simulink model "Hydraulic787"  (R2013a)
settings: Solver=ode23tb  StartTime=0.0  StopTime=1000  RelTol=1e-3
InitFcn:
  | load('SampleOutput.mat')
  | 
  | load('SampleFuelBurn.mat')
undefined symbols (not defined in the file): ailerons, AirProp, B_737, elevator, HydProp, landing_gear, rudder, thrust_rev
libraries: PowerFlowLib x43, simulink x4
(part 2 of 2)

== system Hydraulic787/Center Hydraulic System/DC Speed Servo1 ==
  T_load (Nm) : Inport
  Speed_ref (RPM) : Inport  Port=2
  Voltage : Inport  Port=3
  DC Machine : Subsystem
  Fcn : Fcn  Expr=u(1)/(u(2)+0.1)
  Gain2 : Gain  Gain=60/(2*pi)
  Mux : Mux  Inputs=2
  PID Controller : simulink/Continuous/PID Controller  Controller=PID  TimeDomain=Continuous-time  SampleTime=1  IntegratorMethod=Forward Euler  FilterMethod=Forward Euler  Form=Parallel  P=1  I=0.1  D=0  N=100  InitialConditionSource=internal  InitialConditionForIntegrator=0  InitialConditionForFilter=0  ExternalReset=none  LimitOutput=off  UpperSaturationLimit=inf  LowerSaturationLimit=-inf  LinearizeAsGain=on  AntiWindupMode=none  Kb=1  TrackingMode=off  Kt=1  PParamMin=[]  PParamMax=[]  IParamMin=[]  IParamMax=[]  DParamMin=[]  DParamMax=[]  NParamMin=[]  NParamMax=[]  KbParamMin=[]  KbParamMax=[]  KtParamMin=[]  KtParamMax=[]  POutMin=[]  POutMax=[]  IOutMin=[]  IOutMax=[]  DOutMin=[]  DOutMax=[]  NOutMin=[]  NOutMax=[]  KbOutMin=[]  KbOutMax=[]  KtOutMin=[]  KtOutMax=[]  IntegratorOutMin=[]  IntegratorOutMax=[]  FilterOutMin=[]  FilterOutMax=[]  SumOutMin=[]  SumOutMax=[]  SumI1OutMin=[]  SumI1OutMax=[]  SumI2OutMin=[]  SumI2OutMax=[]  SumI3OutMin=[]  SumI3OutMax=[]  SumDOutMin=[]  SumDOutMax=[]  SaturationOutMin=[]  SaturationOutMax=[]  IntegratorContinuousStateAttributes=''  IntegratorStateMustResolveToSignalObject=off  IntegratorRTWStateStorageClass=Auto  FilterContinuousStateAttributes=''  FilterStateMustResolveToSignalObject=off  FilterRTWStateStorageClass=Auto
  Sum : Sum  Inputs=-+|
  Terminator{,1..3} (4 alike) : Terminator
  w_m : Outport
  i_load : Outport  Port=2
  T_em : Outport  Port=3
  Ploss : Outport  Port=4
  wires:
  DC Machine/5(Plosses) -> Ploss/1
  Sum/1 -> PID Controller/1
  Gain2/1 -> Sum/1, w_m/1
  Speed_ref (RPM)/1 -> Sum/2
  T_load (Nm)/1 -> DC Machine/3(Tload)
  DC Machine/6(Te) -> T_em/1
  Mux/1 -> Fcn/1
  DC Machine/3(Pe) -> Mux/1
  Fcn/1 -> i_load/1
  DC Machine/7(Speed) -> Gain2/1
  Voltage/1 -> DC Machine/1(Vf), Mux/2
  PID Controller/1 -> DC Machine/2(Va)
  DC Machine/1(If) -> Terminator3/1
  DC Machine/2(Ia) -> Terminator2/1
  DC Machine/4(Pm) -> Terminator1/1
  DC Machine/8(theta) -> Terminator/1

== system Hydraulic787/Center Hydraulic System/Sinks ==
  "Motor PLoss 1 " : Inport
  Motor PLoss 2 : Inport  Port=2
  Motor Current Load 1 : Inport  Port=3
  Motor Current Load 2 : Inport  Port=4
  Out1 : Outport
  wires:
  "Motor PLoss 1 "/1 -> Out1/1

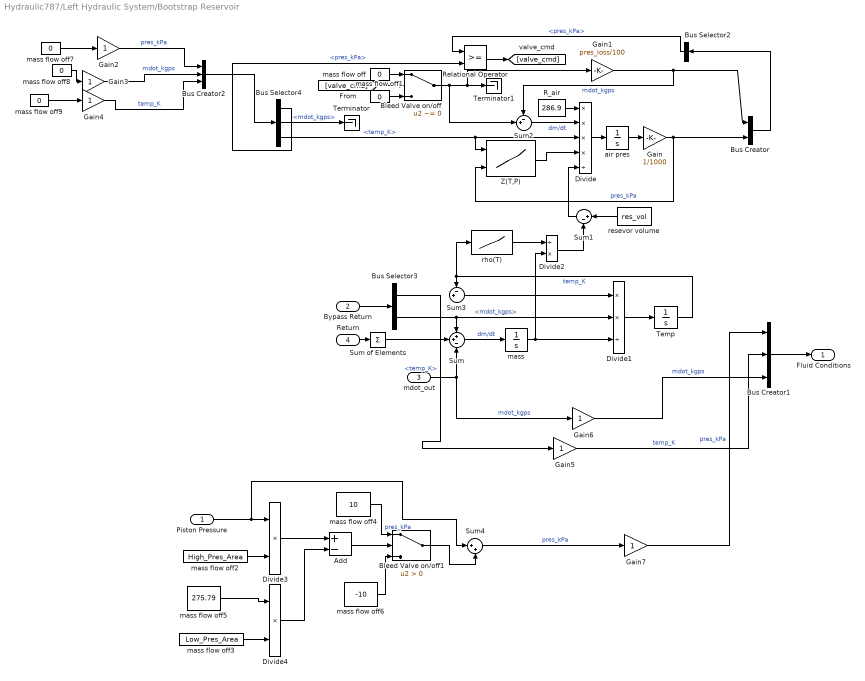
== system Hydraulic787/Left Hydraulic System/Bootstrap Reservoir ==
  Piston Pressure : Inport
  Bypass Return : Inport  Port=2
  mdot_out : Inport  Port=3
  Return : Inport  Port=4
  Add : Sum  Inputs=+-
  Bleed Valve on/off : Switch  Criteria=u2 ~= 0  ZeroCross=off
  Bleed Valve on/off1 : Switch  Criteria=u2 > Threshold  ZeroCross=off
  Bus Creator : BusCreator  Inputs=2
  Bus Creator1 : BusCreator  Inputs=3
  Bus Creator2 : BusCreator  Inputs=3
  Bus Selector2 : BusSelector  OutputSignals=pres_kPa
  Bus Selector3 : BusSelector  OutputSignals=temp_K,mdot_kgps
  Bus Selector4 : BusSelector  OutputSignals=pres_kPa,mdot_kgps,temp_K
  Divide : Product  Inputs=****/
  Divide1 : Product  Inputs=**/
  Divide2 : Product  Inputs=/*
  Divide3 : Product  Inputs=**
  Divide4 : Product  Inputs=**
  Gain : Gain  Gain=1/1000
  Gain1 : Gain  Gain=pres_loss/100
  Gain{2..7} (6 alike) : Gain
  R_air : Constant  Value=286.9
  Relational Operator : RelationalOperator  OutDataTypeStr=boolean
  Sum : Sum  Inputs=++-
  Sum of Elements : Sum  Inputs=+
  Sum1 : Sum  Inputs=|+-
  Sum2 : Sum  Inputs=-+|
  Sum3 : Sum  Inputs=-+|
  Sum4 : Sum  Inputs=|++
  Temp : Integrator  InitialCondition=T_init  LimitOutput=on  LowerSaturationLimit=eps
  Terminator : Terminator
  Terminator1 : Terminator
  Z(T,P) : Lookup_n-D  BreakpointsForDimension1=AirProp.T2  BreakpointsForDimension2=AirProp.P2  Table=AirProp.Z  RndMeth=Simplest  InputSameDT=on
  air pres : Integrator  InitialCondition=P_init*1000
  mass : Integrator  InitialCondition=mass_init  LimitOutput=on  LowerSaturationLimit=eps
  mass flow off{,1,7..9} (5 alike) : Constant  Value=0
  mass flow off2 : Constant  Value=High_Pres_Area
  mass flow off3 : Constant  Value=Low_Pres_Area
  mass flow off4 : Constant  Value=10
  mass flow off5 : Constant  Value=275.79
  mass flow off6 : Constant  Value=-10
  resevor volume : Constant  Value=res_vol
  rho(T) : Lookup_n-D  NumberOfTableDimensions=1  BreakpointsForDimension1=HydProp.T  Table=HydProp.rho_T  RndMeth=Simplest  InputSameDT=on
  Fluid Conditions : Outport
  wires:
  Piston Pressure/1 -> Sum4/1, Divide3/1
  mass flow off1/1 -> Bleed Valve on/off/3
  Divide2/1 -> Sum1/2
  rho(T)/1 -> Divide2/1
  Sum of Elements/1 -> Sum/2
  Return/1 -> Sum of Elements/1
  Bus Selector3/1 -> Gain5/1  "<temp_K>"
  Temp/1 -> rho(T)/1, Sum3/1  "temp_K"
  Sum3/1 -> Divide1/1
  Divide1/1 -> Temp/1
  mass/1 -> Divide1/3, Divide2/2
  Bus Creator1/1 -> Fluid Conditions/1
  [valve_cmd] -> Bleed Valve on/off/2
  Relational Operator/1 -> [valve_cmd]
  mass flow off/1 -> Bleed Valve on/off/1
  Bus Selector2/1 -> Relational Operator/1  "<pres_kPa>"
  Bus Selector4/1 -> Relational Operator/2  "<pres_kPa>"
  Bleed Valve on/off/1 -> Terminator1/1, Gain1/1, Sum2/2
  Bus Selector4/2 -> Terminator/1  "<mdot_kgps>"
  Sum2/1 -> Divide/2  "dm/dt"
  Bus Creator/1 -> Bus Selector2/1
  Gain1/1 -> Sum2/1, Bus Creator/1  "mdot_kgps"
  Gain/1 -> Bus Creator/2, Z(T,P)/2  "pres_kPa"
  Sum1/1 -> Divide/5
  resevor volume/1 -> Sum1/1
  air pres/1 -> Gain/1
  Divide/1 -> air pres/1
  Z(T,P)/1 -> Divide/4
  R_air/1 -> Divide/1
  Bus Selector4/3 -> Divide/3, Z(T,P)/1  "<temp_K>"
  Sum/1 -> mass/1  "dm/dt"
  mdot_out/1 -> Gain6/1, Sum/3  "mdot_kgps"
  Bus Selector3/2 -> Sum/1, Divide1/2  "<mdot_kgps>"
  Bypass Return/1 -> Bus Selector3/1
  mass flow off2/1 -> Divide3/2
  mass flow off3/1 -> Divide4/2
  mass flow off5/1 -> Divide4/1
  Divide4/1 -> Add/2
  Divide3/1 -> Add/1
  Add/1 -> Bleed Valve on/off1/2
  mass flow off6/1 -> Bleed Valve on/off1/3
  Bleed Valve on/off1/1 -> Sum4/2
  mass flow off4/1 -> Bleed Valve on/off1/1  "pres_kPa"
  Bus Creator2/1 -> Bus Selector4/1
  mass flow off9/1 -> Gain4/1
  mass flow off8/1 -> Gain3/1
  mass flow off7/1 -> Gain2/1
  Gain2/1 -> Bus Creator2/1  "pres_kPa"
  Gain4/1 -> Bus Creator2/3  "temp_K"
  Gain3/1 -> Bus Creator2/2  "mdot_kgps"
  Gain7/1 -> Bus Creator1/1  "pres_kPa"
  Gain6/1 -> Bus Creator1/3  "mdot_kgps"
  Gain5/1 -> Bus Creator1/2  "temp_K"
  Sum4/1 -> Gain7/1  "pres_kPa"

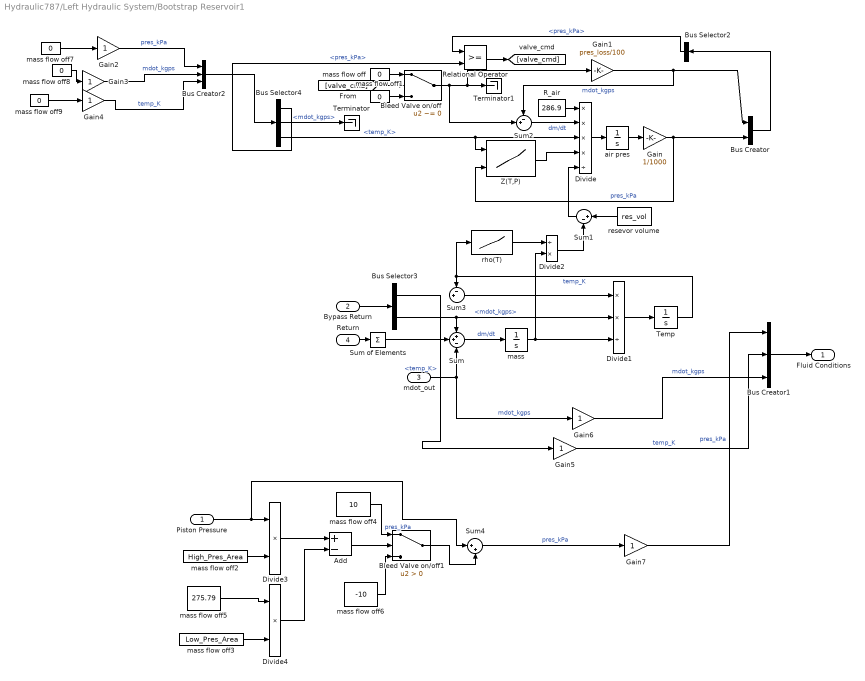
== system Hydraulic787/Left Hydraulic System/Bootstrap Reservoir1 ==
  Piston Pressure : Inport
  Bypass Return : Inport  Port=2
  mdot_out : Inport  Port=3
  Return : Inport  Port=4
  Add : Sum  Inputs=+-
  Bleed Valve on/off : Switch  Criteria=u2 ~= 0  ZeroCross=off
  Bleed Valve on/off1 : Switch  Criteria=u2 > Threshold  ZeroCross=off
  Bus Creator : BusCreator  Inputs=2
  Bus Creator1 : BusCreator  Inputs=3
  Bus Creator2 : BusCreator  Inputs=3
  Bus Selector2 : BusSelector  OutputSignals=pres_kPa
  Bus Selector3 : BusSelector  OutputSignals=temp_K,mdot_kgps
  Bus Selector4 : BusSelector  OutputSignals=pres_kPa,mdot_kgps,temp_K
  Divide : Product  Inputs=****/
  Divide1 : Product  Inputs=**/
  Divide2 : Product  Inputs=/*
  Divide3 : Product  Inputs=**
  Divide4 : Product  Inputs=**
  Gain : Gain  Gain=1/1000
  Gain1 : Gain  Gain=pres_loss/100
  Gain{2..7} (6 alike) : Gain
  R_air : Constant  Value=286.9
  Relational Operator : RelationalOperator  OutDataTypeStr=boolean
  Sum : Sum  Inputs=++-
  Sum of Elements : Sum  Inputs=+
  Sum1 : Sum  Inputs=|+-
  Sum2 : Sum  Inputs=-+|
  Sum3 : Sum  Inputs=-+|
  Sum4 : Sum  Inputs=|++
  Temp : Integrator  InitialCondition=T_init  LimitOutput=on  LowerSaturationLimit=eps
  Terminator : Terminator
  Terminator1 : Terminator
  Z(T,P) : Lookup_n-D  BreakpointsForDimension1=AirProp.T2  BreakpointsForDimension2=AirProp.P2  Table=AirProp.Z  RndMeth=Simplest  InputSameDT=on
  air pres : Integrator  InitialCondition=P_init*1000
  mass : Integrator  InitialCondition=mass_init  LimitOutput=on  LowerSaturationLimit=eps
  mass flow off{,1,7..9} (5 alike) : Constant  Value=0
  mass flow off2 : Constant  Value=High_Pres_Area
  mass flow off3 : Constant  Value=Low_Pres_Area
  mass flow off4 : Constant  Value=10
  mass flow off5 : Constant  Value=275.79
  mass flow off6 : Constant  Value=-10
  resevor volume : Constant  Value=res_vol
  rho(T) : Lookup_n-D  NumberOfTableDimensions=1  BreakpointsForDimension1=HydProp.T  Table=HydProp.rho_T  RndMeth=Simplest  InputSameDT=on
  Fluid Conditions : Outport
  wires:
  Piston Pressure/1 -> Sum4/1, Divide3/1
  mass flow off1/1 -> Bleed Valve on/off/3
  Divide2/1 -> Sum1/2
  rho(T)/1 -> Divide2/1
  Sum of Elements/1 -> Sum/2
  Return/1 -> Sum of Elements/1
  Bus Selector3/1 -> Gain5/1  "<temp_K>"
  Temp/1 -> rho(T)/1, Sum3/1  "temp_K"
  Sum3/1 -> Divide1/1
  Divide1/1 -> Temp/1
  mass/1 -> Divide1/3, Divide2/2
  Bus Creator1/1 -> Fluid Conditions/1
  [valve_cmd] -> Bleed Valve on/off/2
  Relational Operator/1 -> [valve_cmd]
  mass flow off/1 -> Bleed Valve on/off/1
  Bus Selector2/1 -> Relational Operator/1  "<pres_kPa>"
  Bus Selector4/1 -> Relational Operator/2  "<pres_kPa>"
  Bleed Valve on/off/1 -> Terminator1/1, Gain1/1, Sum2/2
  Bus Selector4/2 -> Terminator/1  "<mdot_kgps>"
  Sum2/1 -> Divide/2  "dm/dt"
  Bus Creator/1 -> Bus Selector2/1
  Gain1/1 -> Sum2/1, Bus Creator/1  "mdot_kgps"
  Gain/1 -> Bus Creator/2, Z(T,P)/2  "pres_kPa"
  Sum1/1 -> Divide/5
  resevor volume/1 -> Sum1/1
  air pres/1 -> Gain/1
  Divide/1 -> air pres/1
  Z(T,P)/1 -> Divide/4
  R_air/1 -> Divide/1
  Bus Selector4/3 -> Divide/3, Z(T,P)/1  "<temp_K>"
  Sum/1 -> mass/1  "dm/dt"
  mdot_out/1 -> Gain6/1, Sum/3  "mdot_kgps"
  Bus Selector3/2 -> Sum/1, Divide1/2  "<mdot_kgps>"
  Bypass Return/1 -> Bus Selector3/1
  mass flow off2/1 -> Divide3/2
  mass flow off3/1 -> Divide4/2
  mass flow off5/1 -> Divide4/1
  Divide4/1 -> Add/2
  Divide3/1 -> Add/1
  Add/1 -> Bleed Valve on/off1/2
  mass flow off6/1 -> Bleed Valve on/off1/3
  Bleed Valve on/off1/1 -> Sum4/2
  mass flow off4/1 -> Bleed Valve on/off1/1  "pres_kPa"
  Bus Creator2/1 -> Bus Selector4/1
  mass flow off9/1 -> Gain4/1
  mass flow off8/1 -> Gain3/1
  mass flow off7/1 -> Gain2/1
  Gain2/1 -> Bus Creator2/1  "pres_kPa"
  Gain4/1 -> Bus Creator2/3  "temp_K"
  Gain3/1 -> Bus Creator2/2  "mdot_kgps"
  Gain7/1 -> Bus Creator1/1  "pres_kPa"
  Gain6/1 -> Bus Creator1/3  "mdot_kgps"
  Gain5/1 -> Bus Creator1/2  "temp_K"
  Sum4/1 -> Gain7/1  "pres_kPa"

== system Hydraulic787/Left Hydraulic System/DC Speed Servo ==
  T_load (Nm) : Inport
  Speed_ref (RPM) : Inport  Port=2
  Voltage : Inport  Port=3
  DC Machine : Subsystem
  Fcn : Fcn  Expr=u(1)/(u(2)+0.1)
  Gain2 : Gain  Gain=60/(2*pi)
  Mux : Mux  Inputs=2
  PID Controller : simulink/Continuous/PID Controller  Controller=PID  TimeDomain=Continuous-time  SampleTime=1  IntegratorMethod=Forward Euler  FilterMethod=Forward Euler  Form=Parallel  P=1  I=0.1  D=0  N=100  InitialConditionSource=internal  InitialConditionForIntegrator=0  InitialConditionForFilter=0  ExternalReset=none  LimitOutput=off  UpperSaturationLimit=inf  LowerSaturationLimit=-inf  LinearizeAsGain=on  AntiWindupMode=none  Kb=1  TrackingMode=off  Kt=1  PParamMin=[]  PParamMax=[]  IParamMin=[]  IParamMax=[]  DParamMin=[]  DParamMax=[]  NParamMin=[]  NParamMax=[]  KbParamMin=[]  KbParamMax=[]  KtParamMin=[]  KtParamMax=[]  POutMin=[]  POutMax=[]  IOutMin=[]  IOutMax=[]  DOutMin=[]  DOutMax=[]  NOutMin=[]  NOutMax=[]  KbOutMin=[]  KbOutMax=[]  KtOutMin=[]  KtOutMax=[]  IntegratorOutMin=[]  IntegratorOutMax=[]  FilterOutMin=[]  FilterOutMax=[]  SumOutMin=[]  SumOutMax=[]  SumI1OutMin=[]  SumI1OutMax=[]  SumI2OutMin=[]  SumI2OutMax=[]  SumI3OutMin=[]  SumI3OutMax=[]  SumDOutMin=[]  SumDOutMax=[]  SaturationOutMin=[]  SaturationOutMax=[]  IntegratorContinuousStateAttributes=''  IntegratorStateMustResolveToSignalObject=off  IntegratorRTWStateStorageClass=Auto  FilterContinuousStateAttributes=''  FilterStateMustResolveToSignalObject=off  FilterRTWStateStorageClass=Auto
  Sum : Sum  Inputs=-+|
  Terminator{,1..3} (4 alike) : Terminator
  w_m : Outport
  i_load : Outport  Port=2
  T_em : Outport  Port=3
  Ploss : Outport  Port=4
  wires:
  DC Machine/5(Plosses) -> Ploss/1
  Sum/1 -> PID Controller/1
  Gain2/1 -> Sum/1, w_m/1
  Speed_ref (RPM)/1 -> Sum/2
  T_load (Nm)/1 -> DC Machine/3(Tload)
  DC Machine/6(Te) -> T_em/1
  Mux/1 -> Fcn/1
  DC Machine/3(Pe) -> Mux/1
  Fcn/1 -> i_load/1
  DC Machine/7(Speed) -> Gain2/1
  Voltage/1 -> DC Machine/1(Vf), Mux/2
  PID Controller/1 -> DC Machine/2(Va)
  DC Machine/1(If) -> Terminator/1
  DC Machine/2(Ia) -> Terminator1/1
  DC Machine/4(Pm) -> Terminator2/1
  DC Machine/8(theta) -> Terminator3/1

== system Hydraulic787/Left Hydraulic System/Sinks ==
  "Motor PLoss " : Inport
  Motor Current Load : Inport  Port=2
  Out1 : Outport
  wires:
  "Motor PLoss "/1 -> Out1/1

== system Hydraulic787/Right Hydraulic System/Bootstrap Reservoir ==
  Piston Pressure : Inport
  Bypass Return : Inport  Port=2
  mdot_out : Inport  Port=3
  Return : Inport  Port=4
  Add : Sum  Inputs=+-
  Bleed Valve on/off : Switch  Criteria=u2 ~= 0  ZeroCross=off
  Bleed Valve on/off1 : Switch  Criteria=u2 > Threshold  ZeroCross=off
  Bus Creator : BusCreator  Inputs=2
  Bus Creator1 : BusCreator  Inputs=3
  Bus Creator2 : BusCreator  Inputs=3
  Bus Selector2 : BusSelector  OutputSignals=pres_kPa
  Bus Selector3 : BusSelector  OutputSignals=temp_K,mdot_kgps
  Bus Selector4 : BusSelector  OutputSignals=pres_kPa,mdot_kgps,temp_K
  Divide : Product  Inputs=****/
  Divide1 : Product  Inputs=**/
  Divide2 : Product  Inputs=/*
  Divide3 : Product  Inputs=**
  Divide4 : Product  Inputs=**
  Gain : Gain  Gain=1/1000
  Gain1 : Gain  Gain=pres_loss/100
  Gain{2..7} (6 alike) : Gain
  R_air : Constant  Value=286.9
  Relational Operator : RelationalOperator  OutDataTypeStr=boolean
  Sum : Sum  Inputs=++-
  Sum of Elements : Sum  Inputs=+
  Sum1 : Sum  Inputs=|+-
  Sum2 : Sum  Inputs=-+|
  Sum3 : Sum  Inputs=-+|
  Sum4 : Sum  Inputs=|++
  Temp : Integrator  InitialCondition=T_init  LimitOutput=on  LowerSaturationLimit=eps
  Terminator : Terminator
  Terminator1 : Terminator
  Z(T,P) : Lookup_n-D  BreakpointsForDimension1=AirProp.T2  BreakpointsForDimension2=AirProp.P2  Table=AirProp.Z  RndMeth=Simplest  InputSameDT=on
  air pres : Integrator  InitialCondition=P_init*1000
  mass : Integrator  InitialCondition=mass_init  LimitOutput=on  LowerSaturationLimit=eps
  mass flow off{,1,7..9} (5 alike) : Constant  Value=0
  mass flow off2 : Constant  Value=High_Pres_Area
  mass flow off3 : Constant  Value=Low_Pres_Area
  mass flow off4 : Constant  Value=10
  mass flow off5 : Constant  Value=275.79
  mass flow off6 : Constant  Value=-10
  resevor volume : Constant  Value=res_vol
  rho(T) : Lookup_n-D  NumberOfTableDimensions=1  BreakpointsForDimension1=HydProp.T  Table=HydProp.rho_T  RndMeth=Simplest  InputSameDT=on
  Fluid Conditions : Outport
  wires:
  Piston Pressure/1 -> Sum4/1, Divide3/1
  mass flow off1/1 -> Bleed Valve on/off/3
  Divide2/1 -> Sum1/2
  rho(T)/1 -> Divide2/1
  Sum of Elements/1 -> Sum/2
  Return/1 -> Sum of Elements/1
  Bus Selector3/1 -> Gain5/1  "<temp_K>"
  Temp/1 -> rho(T)/1, Sum3/1  "temp_K"
  Sum3/1 -> Divide1/1
  Divide1/1 -> Temp/1
  mass/1 -> Divide1/3, Divide2/2
  Bus Creator1/1 -> Fluid Conditions/1
  [valve_cmd] -> Bleed Valve on/off/2
  Relational Operator/1 -> [valve_cmd]
  mass flow off/1 -> Bleed Valve on/off/1
  Bus Selector2/1 -> Relational Operator/1  "<pres_kPa>"
  Bus Selector4/1 -> Relational Operator/2  "<pres_kPa>"
  Bleed Valve on/off/1 -> Terminator1/1, Gain1/1, Sum2/2
  Bus Selector4/2 -> Terminator/1  "<mdot_kgps>"
  Sum2/1 -> Divide/2  "dm/dt"
  Bus Creator/1 -> Bus Selector2/1
  Gain1/1 -> Sum2/1, Bus Creator/1  "mdot_kgps"
  Gain/1 -> Bus Creator/2, Z(T,P)/2  "pres_kPa"
  Sum1/1 -> Divide/5
  resevor volume/1 -> Sum1/1
  air pres/1 -> Gain/1
  Divide/1 -> air pres/1
  Z(T,P)/1 -> Divide/4
  R_air/1 -> Divide/1
  Bus Selector4/3 -> Divide/3, Z(T,P)/1  "<temp_K>"
  Sum/1 -> mass/1  "dm/dt"
  mdot_out/1 -> Gain6/1, Sum/3  "mdot_kgps"
  Bus Selector3/2 -> Sum/1, Divide1/2  "<mdot_kgps>"
  Bypass Return/1 -> Bus Selector3/1
  mass flow off2/1 -> Divide3/2
  mass flow off3/1 -> Divide4/2
  mass flow off5/1 -> Divide4/1
  Divide4/1 -> Add/2
  Divide3/1 -> Add/1
  Add/1 -> Bleed Valve on/off1/2
  mass flow off6/1 -> Bleed Valve on/off1/3
  Bleed Valve on/off1/1 -> Sum4/2
  mass flow off4/1 -> Bleed Valve on/off1/1  "pres_kPa"
  Bus Creator2/1 -> Bus Selector4/1
  mass flow off9/1 -> Gain4/1
  mass flow off8/1 -> Gain3/1
  mass flow off7/1 -> Gain2/1
  Gain2/1 -> Bus Creator2/1  "pres_kPa"
  Gain4/1 -> Bus Creator2/3  "temp_K"
  Gain3/1 -> Bus Creator2/2  "mdot_kgps"
  Gain7/1 -> Bus Creator1/1  "pres_kPa"
  Gain6/1 -> Bus Creator1/3  "mdot_kgps"
  Gain5/1 -> Bus Creator1/2  "temp_K"
  Sum4/1 -> Gain7/1  "pres_kPa"

== system Hydraulic787/Right Hydraulic System/Bootstrap Reservoir1 ==
  Piston Pressure : Inport
  Bypass Return : Inport  Port=2
  mdot_out : Inport  Port=3
  Return : Inport  Port=4
  Add : Sum  Inputs=+-
  Bleed Valve on/off : Switch  Criteria=u2 ~= 0  ZeroCross=off
  Bleed Valve on/off1 : Switch  Criteria=u2 > Threshold  ZeroCross=off
  Bus Creator : BusCreator  Inputs=2
  Bus Creator1 : BusCreator  Inputs=3
  Bus Creator2 : BusCreator  Inputs=3
  Bus Selector2 : BusSelector  OutputSignals=pres_kPa
  Bus Selector3 : BusSelector  OutputSignals=temp_K,mdot_kgps
  Bus Selector4 : BusSelector  OutputSignals=pres_kPa,mdot_kgps,temp_K
  Divide : Product  Inputs=****/
  Divide1 : Product  Inputs=**/
  Divide2 : Product  Inputs=/*
  Divide3 : Product  Inputs=**
  Divide4 : Product  Inputs=**
  Gain : Gain  Gain=1/1000
  Gain1 : Gain  Gain=pres_loss/100
  Gain{2..7} (6 alike) : Gain
  R_air : Constant  Value=286.9
  Relational Operator : RelationalOperator  OutDataTypeStr=boolean
  Sum : Sum  Inputs=++-
  Sum of Elements : Sum  Inputs=+
  Sum1 : Sum  Inputs=|+-
  Sum2 : Sum  Inputs=-+|
  Sum3 : Sum  Inputs=-+|
  Sum4 : Sum  Inputs=|++
  Temp : Integrator  InitialCondition=T_init  LimitOutput=on  LowerSaturationLimit=eps
  Terminator : Terminator
  Terminator1 : Terminator
  Z(T,P) : Lookup_n-D  BreakpointsForDimension1=AirProp.T2  BreakpointsForDimension2=AirProp.P2  Table=AirProp.Z  RndMeth=Simplest  InputSameDT=on
  air pres : Integrator  InitialCondition=P_init*1000
  mass : Integrator  InitialCondition=mass_init  LimitOutput=on  LowerSaturationLimit=eps
  mass flow off{,1,7..9} (5 alike) : Constant  Value=0
  mass flow off2 : Constant  Value=High_Pres_Area
  mass flow off3 : Constant  Value=Low_Pres_Area
  mass flow off4 : Constant  Value=10
  mass flow off5 : Constant  Value=275.79
  mass flow off6 : Constant  Value=-10
  resevor volume : Constant  Value=res_vol
  rho(T) : Lookup_n-D  NumberOfTableDimensions=1  BreakpointsForDimension1=HydProp.T  Table=HydProp.rho_T  RndMeth=Simplest  InputSameDT=on
  Fluid Conditions : Outport
  wires:
  Piston Pressure/1 -> Sum4/1, Divide3/1
  mass flow off1/1 -> Bleed Valve on/off/3
  Divide2/1 -> Sum1/2
  rho(T)/1 -> Divide2/1
  Sum of Elements/1 -> Sum/2
  Return/1 -> Sum of Elements/1
  Bus Selector3/1 -> Gain5/1  "<temp_K>"
  Temp/1 -> rho(T)/1, Sum3/1  "temp_K"
  Sum3/1 -> Divide1/1
  Divide1/1 -> Temp/1
  mass/1 -> Divide1/3, Divide2/2
  Bus Creator1/1 -> Fluid Conditions/1
  [valve_cmd] -> Bleed Valve on/off/2
  Relational Operator/1 -> [valve_cmd]
  mass flow off/1 -> Bleed Valve on/off/1
  Bus Selector2/1 -> Relational Operator/1  "<pres_kPa>"
  Bus Selector4/1 -> Relational Operator/2  "<pres_kPa>"
  Bleed Valve on/off/1 -> Terminator1/1, Gain1/1, Sum2/2
  Bus Selector4/2 -> Terminator/1  "<mdot_kgps>"
  Sum2/1 -> Divide/2  "dm/dt"
  Bus Creator/1 -> Bus Selector2/1
  Gain1/1 -> Sum2/1, Bus Creator/1  "mdot_kgps"
  Gain/1 -> Bus Creator/2, Z(T,P)/2  "pres_kPa"
  Sum1/1 -> Divide/5
  resevor volume/1 -> Sum1/1
  air pres/1 -> Gain/1
  Divide/1 -> air pres/1
  Z(T,P)/1 -> Divide/4
  R_air/1 -> Divide/1
  Bus Selector4/3 -> Divide/3, Z(T,P)/1  "<temp_K>"
  Sum/1 -> mass/1  "dm/dt"
  mdot_out/1 -> Gain6/1, Sum/3  "mdot_kgps"
  Bus Selector3/2 -> Sum/1, Divide1/2  "<mdot_kgps>"
  Bypass Return/1 -> Bus Selector3/1
  mass flow off2/1 -> Divide3/2
  mass flow off3/1 -> Divide4/2
  mass flow off5/1 -> Divide4/1
  Divide4/1 -> Add/2
  Divide3/1 -> Add/1
  Add/1 -> Bleed Valve on/off1/2
  mass flow off6/1 -> Bleed Valve on/off1/3
  Bleed Valve on/off1/1 -> Sum4/2
  mass flow off4/1 -> Bleed Valve on/off1/1  "pres_kPa"
  Bus Creator2/1 -> Bus Selector4/1
  mass flow off9/1 -> Gain4/1
  mass flow off8/1 -> Gain3/1
  mass flow off7/1 -> Gain2/1
  Gain2/1 -> Bus Creator2/1  "pres_kPa"
  Gain4/1 -> Bus Creator2/3  "temp_K"
  Gain3/1 -> Bus Creator2/2  "mdot_kgps"
  Gain6/1 -> Bus Creator1/3  "mdot_kgps"
  Gain5/1 -> Bus Creator1/2  "temp_K"
  Sum4/1 -> Gain7/1  "pres_kPa"
  Gain7/1 -> Bus Creator1/1  "pres_kPa"

== system Hydraulic787/Right Hydraulic System/DC Speed Servo ==
  T_load (Nm) : Inport
  Speed_ref (RPM) : Inport  Port=2
  Voltage : Inport  Port=3
  DC Machine : Subsystem
  Fcn : Fcn  Expr=u(1)/(u(2)+0.1)
  Gain2 : Gain  Gain=60/(2*pi)
  Mux : Mux  Inputs=2
  PID Controller : simulink/Continuous/PID Controller  Controller=PID  TimeDomain=Continuous-time  SampleTime=1  IntegratorMethod=Forward Euler  FilterMethod=Forward Euler  Form=Parallel  P=1  I=0.1  D=0  N=100  InitialConditionSource=internal  InitialConditionForIntegrator=0  InitialConditionForFilter=0  ExternalReset=none  LimitOutput=off  UpperSaturationLimit=inf  LowerSaturationLimit=-inf  LinearizeAsGain=on  AntiWindupMode=none  Kb=1  TrackingMode=off  Kt=1  PParamMin=[]  PParamMax=[]  IParamMin=[]  IParamMax=[]  DParamMin=[]  DParamMax=[]  NParamMin=[]  NParamMax=[]  KbParamMin=[]  KbParamMax=[]  KtParamMin=[]  KtParamMax=[]  POutMin=[]  POutMax=[]  IOutMin=[]  IOutMax=[]  DOutMin=[]  DOutMax=[]  NOutMin=[]  NOutMax=[]  KbOutMin=[]  KbOutMax=[]  KtOutMin=[]  KtOutMax=[]  IntegratorOutMin=[]  IntegratorOutMax=[]  FilterOutMin=[]  FilterOutMax=[]  SumOutMin=[]  SumOutMax=[]  SumI1OutMin=[]  SumI1OutMax=[]  SumI2OutMin=[]  SumI2OutMax=[]  SumI3OutMin=[]  SumI3OutMax=[]  SumDOutMin=[]  SumDOutMax=[]  SaturationOutMin=[]  SaturationOutMax=[]  IntegratorContinuousStateAttributes=''  IntegratorStateMustResolveToSignalObject=off  IntegratorRTWStateStorageClass=Auto  FilterContinuousStateAttributes=''  FilterStateMustResolveToSignalObject=off  FilterRTWStateStorageClass=Auto
  Sum : Sum  Inputs=-+|
  Terminator{,1..3} (4 alike) : Terminator
  w_m : Outport
  i_load : Outport  Port=2
  T_em : Outport  Port=3
  Ploss : Outport  Port=4
  wires:
  DC Machine/5(Plosses) -> Ploss/1
  Sum/1 -> PID Controller/1
  Gain2/1 -> Sum/1, w_m/1
  Speed_ref (RPM)/1 -> Sum/2
  T_load (Nm)/1 -> DC Machine/3(Tload)
  DC Machine/6(Te) -> T_em/1
  Mux/1 -> Fcn/1
  DC Machine/3(Pe) -> Mux/1
  Fcn/1 -> i_load/1
  DC Machine/7(Speed) -> Gain2/1
  Voltage/1 -> DC Machine/1(Vf), Mux/2
  PID Controller/1 -> DC Machine/2(Va)
  DC Machine/8(theta) -> Terminator3/1
  DC Machine/1(If) -> Terminator/1
  DC Machine/2(Ia) -> Terminator1/1
  DC Machine/4(Pm) -> Terminator2/1

== system Hydraulic787/Right Hydraulic System/Sinks ==
  "Motor PLoss " : Inport
  Motor Current Load : Inport  Port=2
  Out1 : Outport
  wires:
  "Motor PLoss "/1 -> Out1/1

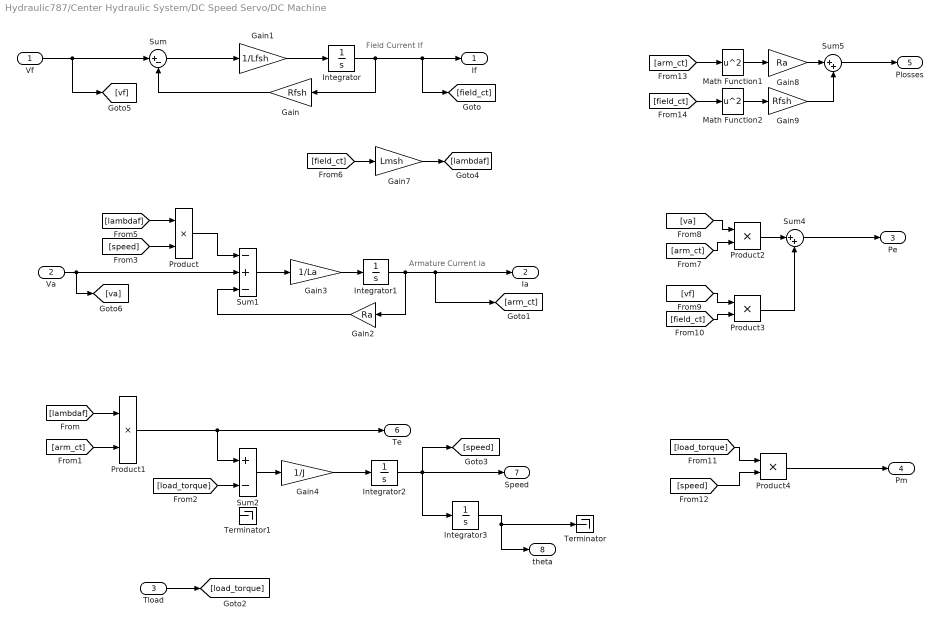
== system Hydraulic787/Center Hydraulic System/DC Speed Servo/DC Machine ==
  note: Armature Current ia
  note: Field Current If
  Vf : Inport
  Va : Inport  Port=2
  Tload : Inport  Port=3
  Gain : Gain  Gain=Rfsh
  Gain1 : Gain  Gain=1/Lfsh
  Gain2 : Gain  Gain=Ra
  Gain3 : Gain  Gain=1/La
  Gain4 : Gain  Gain=1/J
  Gain7 : Gain  Gain=Lmsh
  Gain8 : Gain  Gain=Ra
  Gain9 : Gain  Gain=Rfsh
  Integrator : Integrator
  Integrator1 : Integrator
  Integrator2 : Integrator  InitialCondition=10  LimitOutput=on  LowerSaturationLimit=1
  Integrator3 : Integrator  ZeroCross=off
  Math Function1 : Math  Operator=square  SaturateOnIntegerOverflow=on
  Math Function2 : Math  Operator=square  SaturateOnIntegerOverflow=on
  Product{,1..4} (5 alike) : Product  RndMeth=Zero
  Sum : Sum  Inputs=|+-
  Sum1 : Sum  Inputs=-+-
  Sum2 : Sum  Inputs=+-
  Sum4 : Sum  Inputs=|++
  Sum5 : Sum  Inputs=|++
  Terminator : Terminator
  Terminator1 : Terminator
  If : Outport
  Ia : Outport  Port=2
  Pe : Outport  Port=3
  Pm : Outport  Port=4
  Plosses : Outport  Port=5
  Te : Outport  Port=6
  Speed : Outport  Port=7
  theta : Outport  Port=8
  wires:
  Integrator3/1 -> Terminator/1, theta/1
  Gain/1 -> Sum/2
  Sum/1 -> Gain1/1
  Integrator/1 -> Gain/1, [field_ct], If/1
  Sum1/1 -> Gain3/1
  Gain3/1 -> Integrator1/1
  Integrator1/1 -> Gain2/1, [arm_ct], Ia/1
  Product1/1 -> Sum2/1, Te/1
  Sum2/1 -> Gain4/1
  Gain4/1 -> Integrator2/1
  Gain1/1 -> Integrator/1
  Product/1 -> Sum1/1
  Gain2/1 -> Sum1/3
  [lambdaf] -> Product1/1
  [arm_ct] -> Product1/2
  [load_torque] -> Sum2/2
  [speed] -> Product/2
  [lambdaf] -> Product/1
  [field_ct] -> Gain7/1
  Gain7/1 -> [lambdaf]
  Vf/1 -> Sum/1, [vf]
  Va/1 -> Sum1/2, [va]
  [va] -> Product2/1
  [arm_ct] -> Product2/2
  Product2/1 -> Sum4/1
  [vf] -> Product3/1
  [field_ct] -> Product3/2
  Product3/1 -> Sum4/2
  Sum4/1 -> Pe/1
  [load_torque] -> Product4/1
  [speed] -> Product4/2
  Product4/1 -> Pm/1
  [arm_ct] -> Math Function1/1
  Math Function1/1 -> Gain8/1
  Gain8/1 -> Sum5/1
  [field_ct] -> Math Function2/1
  Math Function2/1 -> Gain9/1
  Gain9/1 -> Sum5/2
  Sum5/1 -> Plosses/1
  Integrator2/1 -> Speed/1, [speed], Integrator3/1
  Tload/1 -> [load_torque]

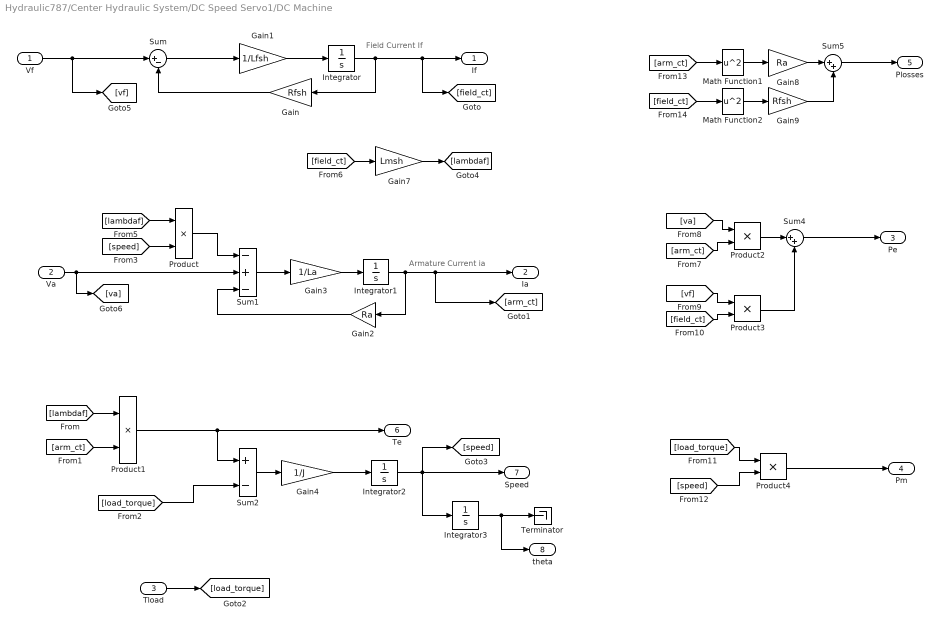
== system Hydraulic787/Center Hydraulic System/DC Speed Servo1/DC Machine ==
  note: Armature Current ia
  note: Field Current If
  Vf : Inport
  Va : Inport  Port=2
  Tload : Inport  Port=3
  Gain : Gain  Gain=Rfsh
  Gain1 : Gain  Gain=1/Lfsh
  Gain2 : Gain  Gain=Ra
  Gain3 : Gain  Gain=1/La
  Gain4 : Gain  Gain=1/J
  Gain7 : Gain  Gain=Lmsh
  Gain8 : Gain  Gain=Ra
  Gain9 : Gain  Gain=Rfsh
  Integrator : Integrator
  Integrator1 : Integrator
  Integrator2 : Integrator  InitialCondition=1  LimitOutput=on  LowerSaturationLimit=1
  Integrator3 : Integrator  ZeroCross=off
  Math Function1 : Math  Operator=square  SaturateOnIntegerOverflow=on
  Math Function2 : Math  Operator=square  SaturateOnIntegerOverflow=on
  Product{,1..4} (5 alike) : Product  RndMeth=Zero
  Sum : Sum  Inputs=|+-
  Sum1 : Sum  Inputs=-+-
  Sum2 : Sum  Inputs=+-
  Sum4 : Sum  Inputs=|++
  Sum5 : Sum  Inputs=|++
  Terminator : Terminator
  If : Outport
  Ia : Outport  Port=2
  Pe : Outport  Port=3
  Pm : Outport  Port=4
  Plosses : Outport  Port=5
  Te : Outport  Port=6
  Speed : Outport  Port=7
  theta : Outport  Port=8
  wires:
  Integrator3/1 -> Terminator/1, theta/1
  Gain/1 -> Sum/2
  Sum/1 -> Gain1/1
  Integrator/1 -> Gain/1, [field_ct], If/1
  Sum1/1 -> Gain3/1
  Gain3/1 -> Integrator1/1
  Integrator1/1 -> Gain2/1, [arm_ct], Ia/1
  Product1/1 -> Sum2/1, Te/1
  Sum2/1 -> Gain4/1
  Gain4/1 -> Integrator2/1
  Gain1/1 -> Integrator/1
  Product/1 -> Sum1/1
  Gain2/1 -> Sum1/3
  [lambdaf] -> Product1/1
  [arm_ct] -> Product1/2
  [load_torque] -> Sum2/2
  [speed] -> Product/2
  [lambdaf] -> Product/1
  [field_ct] -> Gain7/1
  Gain7/1 -> [lambdaf]
  Vf/1 -> Sum/1, [vf]
  Va/1 -> Sum1/2, [va]
  [va] -> Product2/1
  [arm_ct] -> Product2/2
  Product2/1 -> Sum4/1
  [vf] -> Product3/1
  [field_ct] -> Product3/2
  Product3/1 -> Sum4/2
  Sum4/1 -> Pe/1
  [load_torque] -> Product4/1
  [speed] -> Product4/2
  Product4/1 -> Pm/1
  [arm_ct] -> Math Function1/1
  Math Function1/1 -> Gain8/1
  Gain8/1 -> Sum5/1
  [field_ct] -> Math Function2/1
  Math Function2/1 -> Gain9/1
  Gain9/1 -> Sum5/2
  Sum5/1 -> Plosses/1
  Integrator2/1 -> Speed/1, [speed], Integrator3/1
  Tload/1 -> [load_torque]

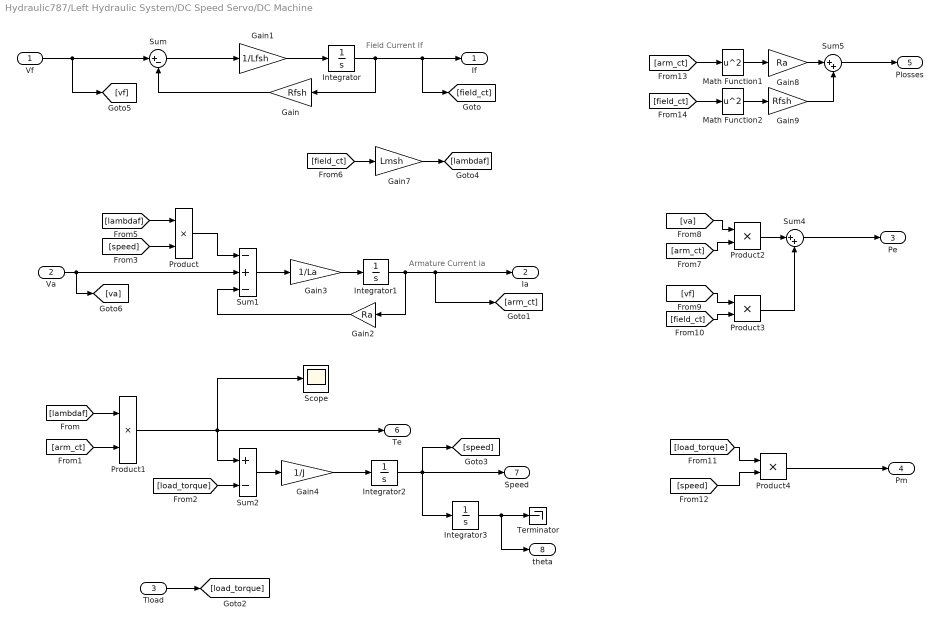
== system Hydraulic787/Left Hydraulic System/DC Speed Servo/DC Machine ==
  note: Armature Current ia
  note: Field Current If
  Vf : Inport
  Va : Inport  Port=2
  Tload : Inport  Port=3
  Gain : Gain  Gain=Rfsh
  Gain1 : Gain  Gain=1/Lfsh
  Gain2 : Gain  Gain=Ra
  Gain3 : Gain  Gain=1/La
  Gain4 : Gain  Gain=1/J
  Gain7 : Gain  Gain=Lmsh
  Gain8 : Gain  Gain=Ra
  Gain9 : Gain  Gain=Rfsh
  Integrator : Integrator
  Integrator1 : Integrator
  Integrator2 : Integrator  InitialCondition=1  LimitOutput=on  LowerSaturationLimit=1
  Integrator3 : Integrator  ZeroCross=off
  Math Function1 : Math  Operator=square  SaturateOnIntegerOverflow=on
  Math Function2 : Math  Operator=square  SaturateOnIntegerOverflow=on
  Product{,1..4} (5 alike) : Product  RndMeth=Zero
  Scope : Scope
      settings: SaveName=ScopeData3
  Sum : Sum  Inputs=|+-
  Sum1 : Sum  Inputs=-+-
  Sum2 : Sum  Inputs=+-
  Sum4 : Sum  Inputs=|++
  Sum5 : Sum  Inputs=|++
  Terminator : Terminator
  If : Outport
  Ia : Outport  Port=2
  Pe : Outport  Port=3
  Pm : Outport  Port=4
  Plosses : Outport  Port=5
  Te : Outport  Port=6
  Speed : Outport  Port=7
  theta : Outport  Port=8
  wires:
  Integrator3/1 -> Terminator/1, theta/1
  Gain/1 -> Sum/2
  Sum/1 -> Gain1/1
  Integrator/1 -> Gain/1, [field_ct], If/1
  Sum1/1 -> Gain3/1
  Gain3/1 -> Integrator1/1
  Integrator1/1 -> Gain2/1, [arm_ct], Ia/1
  Product1/1 -> Scope/1, Sum2/1, Te/1
  Sum2/1 -> Gain4/1
  Gain4/1 -> Integrator2/1
  Gain1/1 -> Integrator/1
  Product/1 -> Sum1/1
  Gain2/1 -> Sum1/3
  [lambdaf] -> Product1/1
  [arm_ct] -> Product1/2
  [load_torque] -> Sum2/2
  [speed] -> Product/2
  [lambdaf] -> Product/1
  [field_ct] -> Gain7/1
  Gain7/1 -> [lambdaf]
  Vf/1 -> Sum/1, [vf]
  Va/1 -> Sum1/2, [va]
  [va] -> Product2/1
  [arm_ct] -> Product2/2
  Product2/1 -> Sum4/1
  [vf] -> Product3/1
  [field_ct] -> Product3/2
  Product3/1 -> Sum4/2
  Sum4/1 -> Pe/1
  [load_torque] -> Product4/1
  [speed] -> Product4/2
  Product4/1 -> Pm/1
  [arm_ct] -> Math Function1/1
  Math Function1/1 -> Gain8/1
  Gain8/1 -> Sum5/1
  [field_ct] -> Math Function2/1
  Math Function2/1 -> Gain9/1
  Gain9/1 -> Sum5/2
  Sum5/1 -> Plosses/1
  Integrator2/1 -> Speed/1, [speed], Integrator3/1
  Tload/1 -> [load_torque]

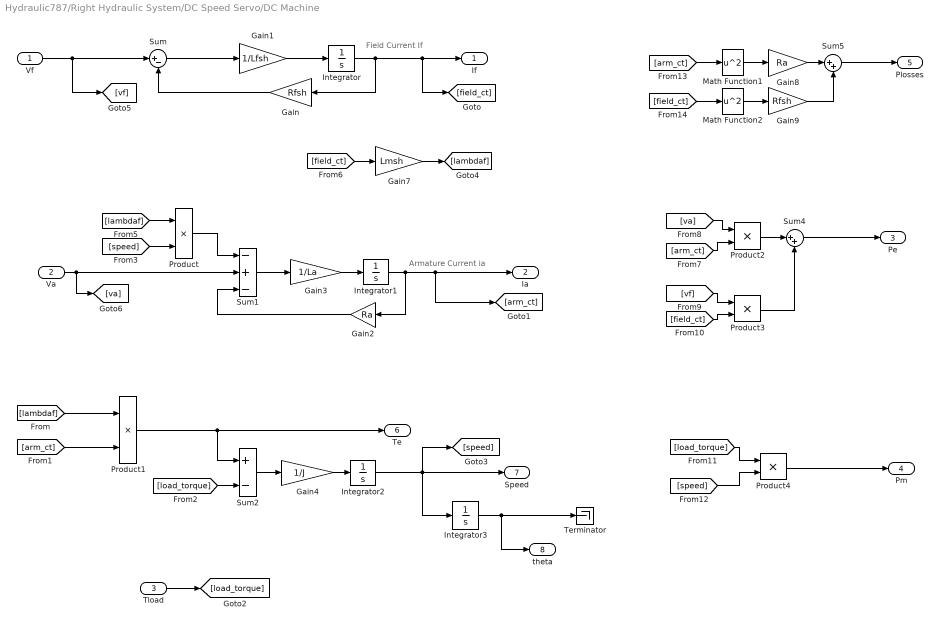
== system Hydraulic787/Right Hydraulic System/DC Speed Servo/DC Machine ==
  note: Armature Current ia
  note: Field Current If
  Vf : Inport
  Va : Inport  Port=2
  Tload : Inport  Port=3
  Gain : Gain  Gain=Rfsh
  Gain1 : Gain  Gain=1/Lfsh
  Gain2 : Gain  Gain=Ra
  Gain3 : Gain  Gain=1/La
  Gain4 : Gain  Gain=1/J
  Gain7 : Gain  Gain=Lmsh
  Gain8 : Gain  Gain=Ra
  Gain9 : Gain  Gain=Rfsh
  Integrator : Integrator
  Integrator1 : Integrator
  Integrator2 : Integrator  InitialCondition=1  LimitOutput=on  LowerSaturationLimit=1
  Integrator3 : Integrator  ZeroCross=off
  Math Function1 : Math  Operator=square  SaturateOnIntegerOverflow=on
  Math Function2 : Math  Operator=square  SaturateOnIntegerOverflow=on
  Product{,1..4} (5 alike) : Product  RndMeth=Zero
  Sum : Sum  Inputs=|+-
  Sum1 : Sum  Inputs=-+-
  Sum2 : Sum  Inputs=+-
  Sum4 : Sum  Inputs=|++
  Sum5 : Sum  Inputs=|++
  Terminator : Terminator
  If : Outport
  Ia : Outport  Port=2
  Pe : Outport  Port=3
  Pm : Outport  Port=4
  Plosses : Outport  Port=5
  Te : Outport  Port=6
  Speed : Outport  Port=7
  theta : Outport  Port=8
  wires:
  Integrator3/1 -> Terminator/1, theta/1
  Gain/1 -> Sum/2
  Sum/1 -> Gain1/1
  Integrator/1 -> Gain/1, [field_ct], If/1
  Sum1/1 -> Gain3/1
  Gain3/1 -> Integrator1/1
  Integrator1/1 -> Gain2/1, [arm_ct], Ia/1
  Product1/1 -> Sum2/1, Te/1
  Sum2/1 -> Gain4/1
  Gain4/1 -> Integrator2/1
  Gain1/1 -> Integrator/1
  Product/1 -> Sum1/1
  Gain2/1 -> Sum1/3
  [lambdaf] -> Product1/1
  [arm_ct] -> Product1/2
  [speed] -> Product/2
  [lambdaf] -> Product/1
  [field_ct] -> Gain7/1
  Gain7/1 -> [lambdaf]
  Vf/1 -> Sum/1, [vf]
  Va/1 -> Sum1/2, [va]
  [va] -> Product2/1
  [arm_ct] -> Product2/2
  Product2/1 -> Sum4/1
  [vf] -> Product3/1
  [field_ct] -> Product3/2
  Product3/1 -> Sum4/2
  Sum4/1 -> Pe/1
  [load_torque] -> Product4/1
  [speed] -> Product4/2
  Product4/1 -> Pm/1
  [arm_ct] -> Math Function1/1
  Math Function1/1 -> Gain8/1
  Gain8/1 -> Sum5/1
  [field_ct] -> Math Function2/1
  Math Function2/1 -> Gain9/1
  Gain9/1 -> Sum5/2
  Sum5/1 -> Plosses/1
  Integrator2/1 -> Speed/1, [speed], Integrator3/1
  Tload/1 -> [load_torque]
  [load_torque] -> Sum2/2
